simulink model "mreset"  (Simulink 6.3)
settings: Solver=ode2  SolverMode=SingleTasking  StartTime=0.0  StopTime=30  FixedStep=1  RelTol=1e-3  AbsTol=1e-6
settings Model: Creator=rajbabu  LastModifiedBy=mshakeri  ExtModeTrigMode=oneshot  ExtModeArmWhenConnect=off  ExtModeAutoUpdateStatusClock=off  StrictBusMsg=None
settings DataIOCC: LimitDataPoints=off  SaveFormat=StructureWithTime  SaveState=on  OutputSaveName=y
settings OptimizationCC: BooleanDataType=off  InlineParams=on  InlineInvariantSignals=on  OptimizeModelRefInitCode=on  LifeSpan=1
settings DebuggingCC: SolverPrmCheckMsg=none  InheritedTsInSrcMsg=none  IntegerOverflowMsg=none
settings HardwareCC: TargetBitPerLong=64  TargetEndianess=LittleEndian  TargetWordSize=64  TargetHWDeviceType=MATLAB Host
settings RTWCC: SystemTargetFile=ert.tlc  TemplateMakefile=ert_default_tmf  Description=Real-Time Workshop Embedded Coder (no auto configuration)  RetainRTWFile=on  ProcessScript=ert_make_rtw_hook
settings CodeAppCC: IgnoreCustomStorageClasses=off
settings ERTTargetCC: TargetFcnLib=ansi_tfl_tmw.mat  GenFloatMathFcnCalls=ANSI_C  GenerateSampleERTMain=on  InlinedParameterPlacement=NonHierarchical  ERTCustomFileTemplate=example_file_process.tlc  InitialValueSource=Model

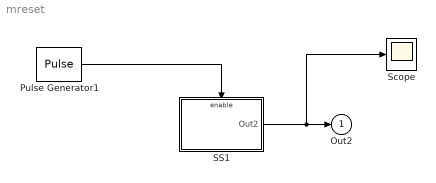
== system mreset ==
  Pulse Generator1 : DiscretePulseGenerator  Period=20  PulseWidth=11
  SS1 : Subsystem
  Scope : Scope
  Out2 : Outport  InitialOutput=0
  wires:
  SS1/1(Out2) -> Out2/1, Scope/1
  Pulse Generator1/1 -> SS1/Enable

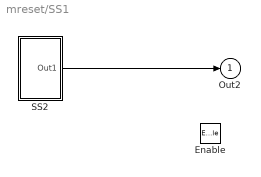
== system mreset/SS1 ==
  Enable : EnablePort  StatesWhenEnabling=reset
  SS2 : Subsystem  TreatAsAtomicUnit=on
  Out2 : Outport  InitialOutput=0
  wires:
  SS2/1(Out1) -> Out2/1

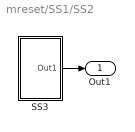
== system mreset/SS1/SS2 ==
  SS3 : Subsystem  TreatAsAtomicUnit=on
  Out1 : Outport
  wires:
  SS3/1(Out1) -> Out1/1

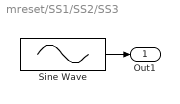
== system mreset/SS1/SS2/SS3 ==
  Sine Wave : Sin  SineType=Sample based  SampleTime=1
  Out1 : Outport
  wires:
  Sine Wave/1 -> Out1/1
